simulink model "Radiator"  (R2016b)
settings: Solver=VariableStepAuto  StartTime=0.0  StopTime=10.0  RelTol=1e-3
model workspace (MATLAB code in the model file):
  | househeat_data_szakdoga
undefined symbols (not defined in the file or in its folder): area_radiator, heat_transfer_const_radiator, supp_water_flow, water_heat_capacity
settings Model: Creator=gylaszlo  LastModifiedBy=gylaszlo

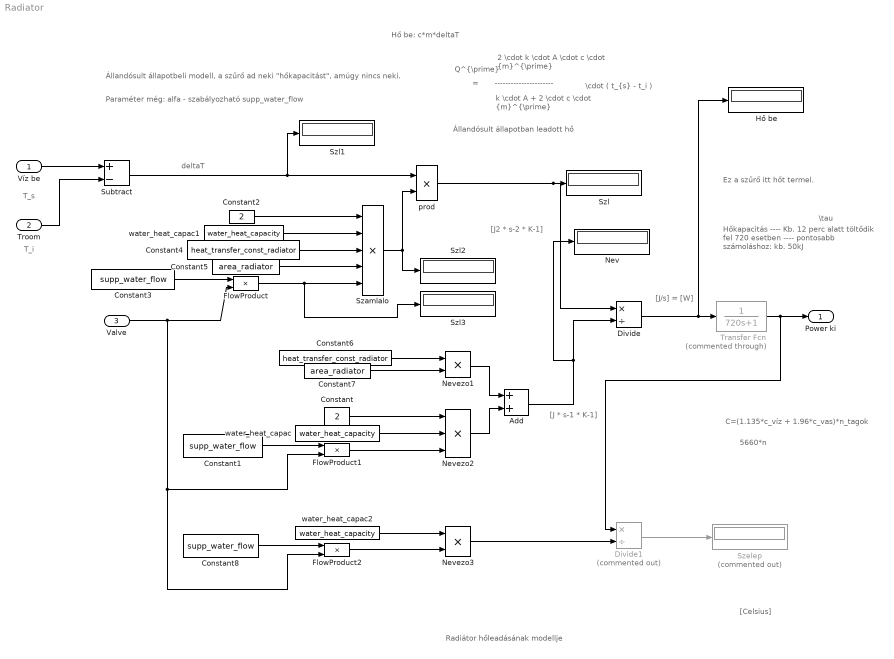
== system Radiator ==
  note: deltaT
  note: Hő be: c*m*deltaT
  note: =
  note: \tau
  note: Ez a szűrő itt hőt termel.
  note: Állandósult állapotban leadott hő
  note: Radiátor hőleadásának modellje
  note: Állandósult állapotbeli modell, a szűrő ad neki "hőkapacitást", amúgy nincs neki.
  note: Paraméter még: alfa - szabályozható supp_water_flow
  note: 5660*n
  note: C=(1.135*c_víz + 1.96*c_vas)*n_tagok
  note: Hőkapacitás
      | ----
      | Kb. 12 perc alatt töltődik fel 720 esetben
      | ----
      | pontosabb számoláshoz: kb. 50kJ
  note: [Celsius]
  note: [J/s] = [W]
  note: [J * s-1 * K-1]
  note: [J2 * s-2 * K-1]
  note: T_i
  note: T_s
  note: ----------------------
  note: =
  note: 2 \cdot k \cdot A \cdot c \cdot {m}^{\prime}
  note: k \cdot A + 2 \cdot c \cdot {m}^{\prime}
  note: \cdot ( t_{s} - t_i )
  note: Q^{\prime}
  Víz be : Inport
  Troom : Inport  Port=2
  Valve : Inport  Port=3
  Add : Sum
  Constant : Constant  Value=2
  Constant1 : Constant  Value=supp_water_flow
  Constant2 : Constant  Value=2
  Constant3 : Constant  Value=supp_water_flow
  Constant4 : Constant  Value=heat_transfer_const_radiator
  Constant5 : Constant  Value=area_radiator
  Constant6 : Constant  Value=heat_transfer_const_radiator
  Constant7 : Constant  Value=area_radiator
  Constant8 : Constant  Value=supp_water_flow
  Divide : Product  Inputs=*/
  Divide1 : Product  Commented=on  Inputs=*/
  FlowProduct : Product
  FlowProduct1 : Product
  FlowProduct2 : Product
  Hő be : Display
  Nev : Display
  Nevezo1 : Product
  Nevezo2 : Product  Inputs=3
  Nevezo3 : Product
  Subtract : Sum  Inputs=+-
  Szamlalo : Product  Inputs=5
  Szelep : Display  Commented=on
  Szl{,1..3} (4 alike) : Display
  Transfer Fcn : TransferFcn  Commented=through  Denominator=[720 1]
  prod : Product  Inputs=**
  water_heat_capac : Constant  Value=water_heat_capacity
  water_heat_capac1 : Constant  Value=water_heat_capacity
  water_heat_capac2 : Constant  Value=water_heat_capacity
  Power ki : Outport
  wires:
  Víz be/1 -> Subtract/1
  Troom/1 -> Subtract/2
  prod/1 -> Divide/1, Szl/1
  Add/1 -> Nev/1, Divide/2
  Nevezo1/1 -> Add/1
  Nevezo2/1 -> Add/2
  Constant/1 -> Nevezo2/1
  water_heat_capac/1 -> Nevezo2/2
  Constant2/1 -> Szamlalo/1
  water_heat_capac1/1 -> Szamlalo/2
  Subtract/1 -> prod/1, Szl1/1
  Constant4/1 -> Szamlalo/3
  Constant5/1 -> Szamlalo/4
  Constant7/1 -> Nevezo1/2
  Constant6/1 -> Nevezo1/1
  Nevezo3/1 -> Divide1/2
  water_heat_capac2/1 -> Nevezo3/1
  Divide1/1 -> Szelep/1
  Transfer Fcn/1 -> Divide1/1, Power ki/1
  Constant3/1 -> FlowProduct/1
  Valve/1 -> FlowProduct2/2, FlowProduct1/2, FlowProduct/2
  FlowProduct1/1 -> Nevezo2/3
  FlowProduct2/1 -> Nevezo3/2
  Constant1/1 -> FlowProduct1/1
  Constant8/1 -> FlowProduct2/1
  Divide/1 -> Hő be/1, Transfer Fcn/1
  FlowProduct/1 -> Szl3/1, Szamlalo/5
  Szamlalo/1 -> Szl2/1, prod/2
